simulink model "Subsystem"  (R2020b)
settings: Solver=VariableStepAuto  StartTime=0.0  StopTime=0.2  RelTol=1e-3
model workspace (MAT data in the model file):
  Kd = Simulink.Parameter
  Kd.Value = 0.15
  Kd.DataType = 'auto'
  Kd.Dimensions = [1 1]
  Ki = Simulink.Parameter
  Ki.Value = 620
  Ki.DataType = 'auto'
  Ki.Dimensions = [1 1]
  Kp = Simulink.Parameter
  Kp.Value = 19
  Kp.DataType = 'auto'
  Kp.Dimensions = [1 1]
  N = Simulink.Parameter
  N.Value = 10000
  N.DataType = 'auto'
  N.Dimensions = [1 1]
settings Model: Creator=hp  LastModifiedBy=hp
settings DataIOCC: SaveOutput=off  SaveTime=off

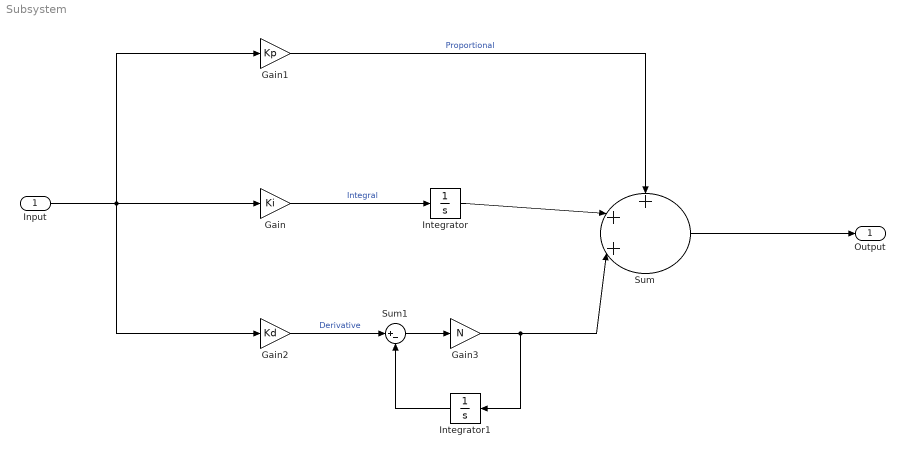
== system Subsystem ==
  Input : Inport  OutDataTypeStr=double  PortDimensions=1  SampleTime=0
  Gain : Gain  Gain=Ki
  Gain1 : Gain  Gain=Kp
  Gain2 : Gain  Gain=Kd
  Gain3 : Gain  Gain=N
  Integrator : Integrator
  Integrator1 : Integrator
  Sum : Sum  Inputs=+++|
  Sum1 : Sum  Inputs=|+-
  Output : Outport  OutDataTypeStr=double  PortDimensions=1  SampleTime=0
  wires:
  Gain3/1 -> Integrator1/1, Sum/3
  Input/1 -> Gain2/1, Gain1/1, Gain/1
  Integrator1/1 -> Sum1/2
  Gain1/1 -> Sum/1  "Proportional"
  Gain/1 -> Integrator/1  "Integral"
  Sum/1 -> Output/1
  Sum1/1 -> Gain3/1
  Gain2/1 -> Sum1/1  "Derivative"
  Integrator/1 -> Sum/2
